simulink model "test3"  (Simulink 6.0)
settings: Solver=ode45  SolverMode=SingleTasking  StartTime=0.0  StopTime=10.0  RelTol=1e-3  AbsTol=1e-6
settings Model: Creator=MD710  LastModifiedBy=MD710
settings DataIOCC: LimitDataPoints=off
settings OptimizationCC: BlockReduction=off  BooleanDataType=off  InlineInvariantSignals=off  InitFltsAndDblsToZero=off
settings DebuggingCC: SolverPrmCheckMsg=none  MultiTaskDSMMsg=warning  MultiTaskCondExecSysMsg=none  FcnCallInpInsideContextMsg=Enable All  StrictBusMsg=None  SFUnexpectedBacktrackingDiag=warning  SFNoUnconditionalDefaultTransitionDiag=warning
settings HardwareCC: TargetHWDeviceType=32-bit Generic  TargetUnknown=on  ProdEqTarget=off
settings RTWCC: IncludeERTFirstTime=on
settings CodeAppCC: CustomSymbolStrType=$N$R$M

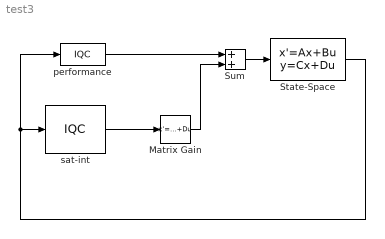
== system test3 ==
  Matrix Gain : StateSpace  A=[]  B=[]  C=[]  D=K  mask(Matrix Gain){K=1}
      mask prompts: K "Gain matrix:"
      mask help: Matrix Gain.
      mask Help: Multiplies input vector by entered matrix to produce output vector (y=Au).
      mask Display: disp('K')
  State-Space : StateSpace  A=[-5,1;2,-3]  B=[0;1]  C=[0 1]  D=[0]
  Sum : Sum  SaturateOnIntegerOverflow=on  InputSameDT=on
  performance : S-Function  FunctionName=IQC  EnableBusSupport=off  mask(IQC block){@1=1, @2=IN=w;OUT=f;}
      mask prompts: @1 "Order"; @2 "List of iqc relationships:"
      mask help: Uncertain blocks specification
      mask Help: IQC block to contain any type of uncertainty
      mask Display: plot(0,0,100,100,[10,20,30,40,30,20,10,0],[50,20,20,50,80,80,50,50],[90,80,70,60,70,80,90,100],[50,20,20,50,80,80,50,50],[55,45],[75,75],[55,45],[65,65],[55,45],[55,55],[46,55],[46,46],[55,46],[35,35],[55,46],[25,25])
  sat-int : S-Function  FunctionName=IQC  EnableBusSupport=off  mask(IQC block){@1=1, @2=out==iqc_ratelimiter(in)}
      mask prompts: @1 "Order"; @2 "List of iqc relationships"
      mask help: Uncertain blocks specification
      mask Help: IQC block to contain any type of uncertainty specified by user
      mask Display: plot(0,0,100,100,[18,45,45,18,18],[60,60,26,26,60],[62,82,82,62,62],[60,60,26,26,60],[62,0],[44,44],[79,65],[44,44],[71,71],[46,57],[68,69,72,74,73,71,69,68,69,72,74],[31,29,29,31,34,35,36,38,40,40,39],[31,31],[26,60],[45,38,24],[55,55,33],[24,18],[33,33],[99,82],[44,44],[10,12,8,10,10,90,90],[44,51,51,44,80,80,44],[7,2],[55,55])
  wires:
  Sum/1 -> State-Space/1
  Matrix Gain/1 -> Sum/2
  performance/1 -> Sum/1
  State-Space/1 -> performance/1, sat-int/1
  sat-int/1 -> Matrix Gain/1
